simulink model "DOB_MSD_poleplace_sim"  (R2020b)
settings: Solver=VariableStepAuto  StartTime=0.0  StopTime=10.0  RelTol=1e-3
values from neighbouring files (symbols this model uses):
  A = [A0 b zeros(n0,1);zeros(1,n0) 0 0; zeros(1,n0) 0 Aa]    [DOB_MSD_LMI_Ptn1.m]    (also in DOB_MSD_poleplace.m = [A0 b ;zeros(1,n0) 0]; Hinf_DOB_MSD_LMI.m)
  B = [b; 0]    [DOB_MSD_poleplace.m]
  C = [c 0]    [DOB_MSD_poleplace.m]
  L = inv(U1) * inv(Y_U_a)*N_a    [DOB_MSD_LMI_Ptn1.m]    (also in DOB_MSD_poleplace.m = -place(A',C',p)'; Hinf_DOB_MSD_LMI.m)
libraries: cstblocks x2
settings Model: Creator=s0612  LastModifiedBy=s0612

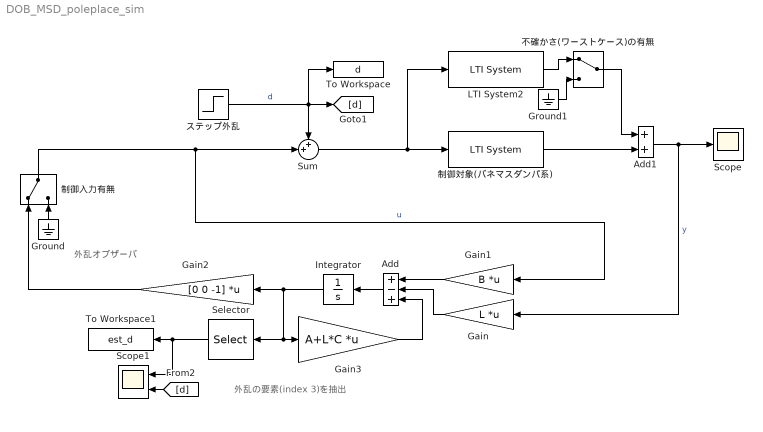
== system DOB_MSD_poleplace_sim ==
  note: 外乱オブザーバ
  note: 外乱の要素(index 3)を抽出
  Add : Sum  Inputs=+-+
  Add1 : Sum
  Gain : Gain  Gain=L  Multiplication=Matrix(K*u) (u vector)
  Gain1 : Gain  Gain=B  Multiplication=Matrix(K*u) (u vector)
  Gain2 : Gain  Gain=[0 0 -1]  Multiplication=Matrix(K*u) (u vector)
  Gain3 : Gain  Gain=A+L*C  Multiplication=Matrix(K*u) (u vector)
  Ground : Ground
  Ground1 : Ground
  Integrator : Integrator
  LTI System2 : cstblocks/LTI System  sys=Wa  IC=[]
  Scope : Scope
  Scope1 : Scope  NumInputPorts=2
  Selector : Selector  InputPortWidth=3  IndexOptions=Index vector (dialog)  Indices=[3]  OutputSizes=1
  Sum : Sum  Inputs=++|
  To Workspace : ToWorkspace  VariableName=d  SaveFormat=Timeseries  SampleTime=-1
  To Workspace1 : ToWorkspace  VariableName=est_d  SaveFormat=Timeseries  SampleTime=-1
  ステップ外乱 : Step  SampleTime=0
  不確かさ(ワーストケース)の有無 : ManualSwitch
  制御入力有無 : ManualSwitch
  制御対象(バネマスダンパ系) : cstblocks/LTI System  sys=P  IC=[]
  wires:
  Add/1 -> Integrator/1
  Integrator/1 -> Selector/1, Gain3/1, Gain2/1
  Gain3/1 -> Add/3
  Gain1/1 -> Add/1
  [d] -> Scope1/2
  Gain/1 -> Add/2
  制御入力有無/1 -> Gain1/1, Sum/2  "u"
  ステップ外乱/1 -> To Workspace/1, [d], Sum/1  "d"
  Sum/1 -> LTI System2/1, 制御対象(バネマスダンパ系)/1
  Add1/1 -> Gain/1, Scope/1  "y"
  Gain2/1 -> 制御入力有無/1
  Selector/1 -> To Workspace1/1, Scope1/1
  不確かさ(ワーストケース)の有無/1 -> Add1/1
  LTI System2/1 -> 不確かさ(ワーストケース)の有無/1
  制御対象(バネマスダンパ系)/1 -> Add1/2
  Ground/1 -> 制御入力有無/2
  Ground1/1 -> 不確かさ(ワーストケース)の有無/2
